simulink model "SimulinkAnalysisofCheetahTail"  (R2022a)
settings: Solver=ode4  StartTime=0.0  StopTime=1.5  FixedStep=0.001  RelTol=1e-3
undefined symbols (not defined in the file): B_cg_H, B_con_H, B_con_L, bar_len, cd_table, Cf, cl_table, g, gear_ratio, int_point_bar, int_point_tail, ITail, M_add, M_cg_H, M_cg_L, M_cg_W, Mb, Mm, Mt, psi3, rho, T_cg_H, T_fur_gap, T_length, T_width_major, T_width_minor, th2_initial, torque_constant, uncertainty_Forces, uncertainty_Position, Vf, windspeed
(part 16 of 21)

== matlab function SimulinkAnalysisofCheetahTail/Model/Forces/NonConstraintForceMatrix_tail_5 ==
  data: B_con_H parameter; B_con_L parameter; Cd input; Cl input; M_cg_H parameter; M_cg_L parameter; M_cg_W parameter; T_fur_gap parameter; T_length parameter; T_width_major parameter; T_width_minor parameter; area_tail_5_drag input; bar_len parameter; int_point_tail input; psi3 parameter; rho parameter; windspeed parameter; q input; dq input; ddq input; Q_tail_5 output
function Q_tail_5 = NonConstraintForceMatrix_tail_5(B_con_H,B_con_L,Cd,Cl,M_cg_H,M_cg_L,M_cg_W,T_fur_gap,T_length,T_width_major,T_width_minor,area_tail_5_drag,bar_len,int_point_tail,psi3,rho,windspeed,q,dq,ddq)
%#codegen
[x,y,z,phi1,th1,psi1,phi2,th2] = deal(q(1),q(2),q(3),q(4),q(5),q(6),q(7),q(8));
[dx,dy,dz,dphi1,dth1,dpsi1,dphi2,dth2] = deal(dq(1),dq(2),dq(3),dq(4),dq(5),dq(6),dq(7),dq(8));
[ddx,ddy,ddz,ddphi1,ddth1,ddpsi1,ddphi2,ddth2] = deal(ddq(1),ddq(2),ddq(3),ddq(4),ddq(5),ddq(6),ddq(7),ddq(8));
%    This function was generated by the Symbolic Math Toolbox version 9.0.
%    17-Feb-2022 12:30:45

t2 = cos(phi1);
t3 = cos(phi2);
t4 = cos(psi1);
t5 = cos(psi3);
t6 = cos(th1);
t7 = cos(th2);
t8 = sin(phi1);
t9 = sin(phi2);
t10 = sin(psi1);
t11 = sin(psi3);
t12 = sin(th1);
t13 = sin(th2);
t14 = M_cg_L+x;
t15 = M_cg_W+y;
t16 = M_cg_H+z;
t19 = -int_point_tail;
t45 = T_length.*(9.0./1.0e+1);
t46 = bar_len.*(9.0./1.0e+1);
t47 = int_point_tail.*(9.0./1.0e+1);
t17 = B_con_L.*t6;
t18 = B_con_L.*t12;
t20 = t2.*t4;
t21 = t6.*t7;
t22 = t2.*t10;
t23 = t4.*t8;
t24 = t7.*t12;
t25 = t8.*t10;
t26 = t12.*t13;
t27 = B_con_H.*t2.*t6;
t29 = t6.*t14;
t30 = B_con_H.*t2.*t12;
t31 = B_con_H.*t6.*t8;
t34 = t12.*t14;
t38 = t6.*t9.*t13;
t40 = t6.*t10.*t13;
t42 = t8.*t9.*t12;
t48 = t2.*t3.*t6;
t49 = T_length+bar_len+t19;
t52 = t2.*t6.*t9;
t53 = t3.*t6.*t8;
t55 = t2.*t6.*t13;
t56 = t3.*t6.*t13;
t58 = t4.*t6.*t13;
t61 = t3.*t8.*t12;
t62 = t6.*t8.*t9;
t67 = t2.*t6.*t15;
t69 = t2.*t6.*t16;
t72 = t6.*t8.*t15;
t73 = t2.*t12.*t16;
t74 = t6.*t8.*t16;
t76 = t8.*t12.*t15;
t79 = -t47;
t105 = t5.*t6.*t8.*t13;
t111 = t6.*t8.*t11.*t13;
t28 = t4.*t17;
t32 = t4.*t18;
t33 = t10.*t17;
t35 = t10.*t18;
t36 = t2.*t26;
t37 = t3.*t26;
t39 = t9.*t24;
t41 = t10.*t24;
t43 = t12.*t25;
t44 = t9.*t26;
t50 = t2.*t21;
t51 = t4.*t21;
t54 = t12.*t20;
t57 = t3.*t24;
t59 = t4.*t24;
t60 = t10.*t21;
t63 = t12.*t22;
t64 = t12.*t23;
t65 = B_con_H.*t6.*t20;
t66 = t4.*t29;
t68 = B_con_H.*t6.*t22;
t70 = t4.*t34;
t71 = t10.*t29;
t75 = t10.*t34;
t77 = -t30;
t78 = -t31;
t81 = -t42;
t86 = t3.*t6.*t23;
t87 = t13.*t48;
t90 = t3.*t8.*t21;
t91 = t6.*t13.*t20;
t92 = t4.*t56;
t95 = t3.*t6.*t25;
t96 = t6.*t9.*t23;
t97 = t2.*t38;
t99 = t8.*t9.*t21;
t100 = t6.*t13.*t22;
t102 = t3.*t40;
t103 = t4.*t38;
t106 = t6.*t9.*t25;
t110 = t10.*t38;
t113 = -t58;
t116 = t6.*t16.*t20;
t117 = t6.*t15.*t23;
t118 = t6.*t16.*t22;
t119 = t6.*t15.*t25;
t120 = -t67;
t121 = -t72;
t122 = -t73;
t123 = -t74;
t124 = t3.*t20.*t21;
t125 = t3.*t21.*t22;
t126 = t9.*t20.*t21;
t127 = t9.*t21.*t22;
t133 = -t105;
t138 = t24+t55;
t226 = t45+t46+t79;
t80 = -t36;
t82 = -t43;
t83 = -t44;
t84 = t3.*t50;
t85 = t3.*t51;
t88 = t2.*t57;
t89 = t9.*t50;
t93 = t3.*t60;
t94 = t9.*t51;
t98 = t2.*t39;
t101 = t4.*t37;
t104 = t9.*t60;
t107 = -t50;
t108 = t10.*t37;
t109 = t4.*t44;
t112 = -t54;
t114 = -t60;
t115 = t10.*t44;
t129 = -t92;
t131 = -t99;
t136 = -t117;
t137 = -t119;
t139 = t22+t64;
t140 = t23+t63;
t141 = -t124;
t142 = -t125;
t149 = t5.*t138;
t153 = t11.*t138;
t157 = t52+t90;
t161 = t57+t87;
t162 = t59+t91;
t163 = t39+t97;
t164 = t41+t100;
t128 = -t84;
t130 = -t93;
t132 = -t104;
t134 = t4.*t83;
t135 = t10.*t83;
t143 = B_con_H.*t139;
t144 = B_con_H.*t140;
t145 = t21+t80;
t146 = t26+t107;
t147 = t20+t82;
t148 = t25+t112;
t150 = t3.*t139;
t151 = t3.*t140;
t152 = t7.*t140;
t154 = t9.*t139;
t155 = t9.*t140;
t156 = t13.*t140;
t165 = t15.*t139;
t166 = t15.*t140;
t167 = t16.*t139;
t168 = t16.*t140;
t174 = t5.*t13.*t139;
t176 = t11.*t13.*t139;
t184 = -t153;
t188 = t48+t131;
t189 = T_fur_gap.*t157;
t190 = T_fur_gap.*t161;
t191 = int_point_tail.*t157;
t192 = int_point_tail.*t161;
t199 = t5.*t162;
t200 = t11.*t162;
t201 = t5.*t163;
t202 = t5.*t164;
t203 = t11.*t163;
t204 = t11.*t164;
t228 = t38+t61+t98;
t231 = t56+t81+t88;
t232 = t53+t83+t89;
t266 = t96+t101+t141;
t268 = t106+t108+t142;
t295 = t157.*t226;
t296 = t161.*t226;
t158 = B_con_H.*t147;
t159 = B_con_H.*t148;
t160 = -t144;
t169 = t7.*t150;
t170 = t7.*t151;
t171 = t13.*t151;
t172 = t7.*t154;
t173 = t9.*t152;
t175 = t13.*t155;
t177 = t5.*t145;
t178 = t5.*t146;
t179 = t3.*t147;
t180 = t3.*t148;
t181 = t7.*t148;
t182 = t11.*t145;
t183 = t11.*t146;
t185 = t9.*t147;
t186 = t9.*t148;
t187 = t13.*t148;
t193 = t15.*t147;
t194 = t15.*t148;
t195 = -t166;
t196 = t16.*t147;
t197 = t16.*t148;
t198 = -t168;
t211 = t5.*t13.*t147;
t213 = t11.*t13.*t147;
t214 = -t176;
t220 = t5.*t188;
t221 = t11.*t188;
t222 = -t204;
t227 = t40+t152;
t229 = t114+t156;
t230 = t37+t62+t128;
t236 = t5.*t228;
t237 = t11.*t228;
t239 = T_fur_gap.*t231;
t240 = T_fur_gap.*t232;
t242 = int_point_tail.*t231;
t243 = int_point_tail.*t232;
t246 = -t5.*(t60-t156);
t249 = -t11.*(t60-t156);
t250 = t5.*t232;
t252 = t11.*t232;
t267 = t86+t126+t134;
t269 = t95+t127+t135;
t276 = T_fur_gap.*t266;
t277 = int_point_tail.*t266;
t278 = T_fur_gap.*t268;
t279 = int_point_tail.*t268;
t317 = t226.*t231;
t318 = t226.*t232;
t345 = t226.*t266;
t347 = t226.*t268;
t370 = t190+t192+t296;
t397 = t78+t120+t123+t189+t191+t295;
t205 = t7.*t179;
t206 = t7.*t180;
t207 = -t169;
t208 = t13.*t180;
t209 = t7.*t185;
t210 = t9.*t181;
t212 = t13.*t186;
t215 = -t177;
t216 = -t179;
t217 = -t183;
t218 = -t193;
t219 = -t194;
t225 = -t213;
t233 = t51+t187;
t234 = t5.*t227;
t235 = t11.*t227;
t238 = T_fur_gap.*t230;
t241 = int_point_tail.*t230;
t244 = t113+t181;
t251 = t12.*t230;
t254 = t130+t171;
t256 = t132+t175;
t257 = t2.*t6.*t230;
t258 = -t5.*(t58-t181);
t259 = t6.*t8.*t230;
t260 = -t11.*(t58-t181);
t262 = -T_fur_gap.*(t93-t171);
t264 = -int_point_tail.*(t93-t171);
t265 = t111+t220;
t270 = -t5.*(t104-t175);
t272 = -t11.*(t104-t175);
t274 = t5.*(t58-t181);
t280 = t133+t221;
t281 = t5.*t269;
t282 = t11.*t269;
t283 = t5.*t267;
t284 = t11.*t267;
t286 = t172+t180;
t288 = t178+t203;
t298 = -T_fur_gap.*(t169-t186);
t300 = -int_point_tail.*(t169-t186);
t302 = t149+t252;
t303 = t102+t170+t185;
t304 = t182+t236;
t308 = t184+t250;
t314 = t226.*t230;
t329 = -t12.*(t153-t250);
t335 = -t2.*t6.*(t153-t250);
t336 = -t6.*t8.*(t153-t250);
t342 = -t226.*(t93-t171);
t344 = t2.*t6.*(t153-t250);
t359 = -t226.*(t169-t186);
t395 = t240+t243+t318;
t396 = t230.*t370;
t401 = -t370.*(t153-t250);
t402 = t370.*(t153-t250);
t404 = -t230.*(t31+t67+t74-t189-t191-t295);
t412 = t17+t29+t76+t77+t122+t239+t242+t317;
t417 = (t153-t250).*(t31+t67+t74-t189-t191-t295);
t432 = t35+t68+t75+t118+t137+t278+t279+t347;
t433 = t32+t65+t70+t116+t136+t276+t277+t345;
t223 = -t205;
t224 = -t210;
t245 = t5.*t233;
t247 = t11.*t233;
t248 = -t234;
t253 = t85+t208;
t255 = t94+t212;
t273 = -t257;
t285 = t151+t209;
t287 = -t283;
t290 = t186+t207;
t292 = t5.*t286;
t294 = t11.*t286;
t301 = t201+t217;
t305 = T_fur_gap.*t303;
t306 = int_point_tail.*t303;
t307 = t129+t154+t206;
t310 = t215+t237;
t311 = t110+t173+t216;
t312 = t12.*t302;
t315 = t5.*t303.*windspeed;
t323 = t2.*t6.*t302;
t324 = t6.*t8.*t302;
t325 = t6.*t10.*t303;
t346 = t199+t284;
t348 = t202+t282;
t350 = t222+t281;
t352 = t140.*t303;
t353 = t235+t270;
t357 = t147.*t303;
t365 = t226.*t303;
t399 = t262+t264+t342;
t400 = t302.*t370;
t403 = t230.*t395;
t411 = t18+t27+t34+t69+t121+t238+t241+t314;
t413 = t302.*t395;
t414 = -t302.*(t31+t67+t74-t189-t191-t295);
t416 = -t395.*(t153-t250);
t418 = t395.*(t153-t250);
t424 = -t417;
t427 = -t303.*(T_fur_gap.*(t93-t171)+int_point_tail.*(t93-t171)+t226.*(t93-t171));
t431 = t303.*(T_fur_gap.*(t93-t171)+int_point_tail.*(t93-t171)+t226.*(t93-t171));
t439 = t230.*t412;
t452 = t302.*t412;
t453 = -t412.*(t153-t250);
t455 = t412.*(t153-t250);
t456 = t143+t167+t219+t298+t300+t359;
t462 = t303.*t432;
t261 = T_fur_gap.*t253;
t263 = int_point_tail.*t253;
t271 = t11.*t255;
t275 = t5.*t255;
t289 = t155+t223;
t291 = t5.*t285;
t293 = t11.*t285;
t309 = t103+t150+t224;
t313 = T_fur_gap.*t307;
t319 = int_point_tail.*t307;
t320 = T_fur_gap.*t311;
t322 = int_point_tail.*t311;
t327 = t5.*t311;
t330 = t11.*t311;
t332 = t11.*t307.*windspeed;
t333 = t19.*t307;
t334 = t4.*t6.*t307;
t337 = -t324;
t341 = t226.*t253;
t349 = t200+t287;
t351 = t174+t294;
t354 = t214+t292;
t356 = t139.*t307;
t360 = t248+t272;
t362 = t148.*t307;
t366 = t226.*t307;
t368 = t226.*t311;
t406 = -t403;
t422 = t157.*t411;
t423 = t161.*t411;
t428 = t231.*t411;
t429 = t232.*t411;
t434 = t5.*t230.*t411;
t435 = t11.*t230.*t411;
t441 = -t439;
t444 = t265.*t411;
t445 = -t411.*(t105-t221);
t447 = t288.*t411;
t448 = -t411.*(t183-t201);
t450 = t304.*t411;
t451 = -t411.*(t177-t237);
t454 = -t452;
t463 = t307.*t433;
t476 = t33+t71+t160+t198+t218+t305+t306+t365;
t481 = -t307.*(-t143-t167+t194+T_fur_gap.*(t169-t186)+int_point_tail.*(t169-t186)+t226.*(t169-t186));
t490 = t307.*(-t143-t167+t194+T_fur_gap.*(t169-t186)+int_point_tail.*(t169-t186)+t226.*(t169-t186));
t297 = T_fur_gap.*t289;
t299 = int_point_tail.*t289;
t316 = T_fur_gap.*t309;
t321 = int_point_tail.*t309;
t326 = t5.*t309;
t328 = t11.*t309;
t331 = -t313;
t338 = -t327;
t340 = -t332;
t343 = -t334;
t355 = t211+t293;
t358 = t226.*t289;
t361 = t225+t291;
t363 = t260+t275;
t364 = t271+t274;
t367 = t226.*t309;
t369 = -t366;
t372 = t246+t330;
t375 = t5.*windspeed.*(t330-t5.*(t60-t156));
t378 = t6.*t10.*(t330-t5.*(t60-t156));
t379 = -t5.*windspeed.*(t327+t11.*(t60-t156));
t384 = -t6.*t10.*(t327+t11.*(t60-t156));
t388 = t140.*(t330-t5.*(t60-t156));
t391 = t147.*(t330-t5.*(t60-t156));
t392 = -t140.*(t327+t11.*(t60-t156));
t394 = -t147.*(t327+t11.*(t60-t156));
t398 = t261+t263+t341;
t415 = t259+t356+t357;
t421 = t273+t352+t362;
t436 = -t428;
t437 = -t429;
t440 = -t435;
t443 = t320+t322+t368;
t446 = -t444;
t449 = -t447;
t459 = -(t330-t5.*(t60-t156)).*(T_fur_gap.*(t93-t171)+int_point_tail.*(t93-t171)+t226.*(t93-t171));
t461 = (t327+t11.*(t60-t156)).*(T_fur_gap.*(t93-t171)+int_point_tail.*(t93-t171)+t226.*(t93-t171));
t465 = -t463;
t492 = t432.*(t330-t5.*(t60-t156));
t496 = -t432.*(t327+t11.*(t60-t156));
t506 = -t476.*(t93-t171);
t507 = t476.*(t93-t171);
t508 = t268.*t476;
t510 = t289.*t476;
t518 = t5.*t303.*t476;
t519 = t11.*t303.*t476;
t520 = t311.*t476;
t522 = t348.*t476;
t524 = -t476.*(t204-t281);
t528 = t353.*t476;
t530 = -t476.*(t234+t11.*(t104-t175));
t532 = -t476.*(t213-t291);
t339 = -t328;
t371 = t247+t326;
t374 = t249+t338;
t385 = -t378;
t405 = t251+t325+t343;
t419 = ddy.*t415;
t420 = dy.*t415;
t425 = ddz.*t421;
t426 = dz.*t421;
t430 = t307.*t398;
t442 = t316+t321+t367;
t458 = t158+t195+t196+t297+t299+t358;
t464 = t303.*t443;
t478 = t28+t66+t159+t165+t197+t331+t333+t369;
t497 = -t492;
t500 = t443.*(t330-t5.*(t60-t156));
t502 = -t443.*(t327+t11.*(t60-t156));
t512 = -t510;
t521 = -t519;
t529 = t355.*t476;
t531 = -t528;
t373 = t245+t339;
t376 = t11.*t371.*windspeed;
t377 = t4.*t6.*t371;
t387 = t139.*t371;
t389 = t148.*t371;
t407 = ddx.*t405;
t408 = dx.*t405;
t438 = -t430;
t457 = t371.*t398;
t466 = t307.*t442;
t482 = t303.*t458;
t493 = t371.*t433;
t501 = t371.*t442;
t509 = t253.*t478;
t511 = t266.*t478;
t513 = -t371.*(-t143-t167+t194+T_fur_gap.*(t169-t186)+int_point_tail.*(t169-t186)+t226.*(t169-t186));
t515 = t458.*(t330-t5.*(t60-t156));
t516 = -t458.*(t327+t11.*(t60-t156));
t517 = -t478.*(t169-t186);
t523 = t309.*t478;
t525 = t5.*t307.*t478;
t526 = t11.*t307.*t478;
t533 = -t529;
t534 = t346.*t478;
t535 = t349.*t478;
t536 = t351.*t478;
t538 = -t478.*(t176-t292);
t539 = t478.*(t176-t292);
t540 = t363.*t478;
t541 = t364.*t478;
Q_tail_5 = ft_1({Cd,Cl,T_fur_gap,T_width_major,T_width_minor,area_tail_5_drag,ddphi1,ddphi2,ddth1,ddth2,ddx,ddy,ddz,dphi1,dphi2,dth1,dth2,dx,dy,dz,int_point_tail,rho,t10,t104,t105,t11,t12,t138,t139,t140,t143,t147,t148,t153,t156,t167,t169,t171,t175,t177,t186,t189,t191,t194,t2,t204,t213,t221,t226,t230,t232,t233,t234,t237,t250,t281,t291,t295,t302,t303,t307,t309,t31,t311,t312,t315,t323,t327,t329,t330,t332,t336,t337,t340,t344,t370,t371,t373,t375,t376,t377,t379,t384,t385,t387,t388,t389,t391,t392,t394,t395,t396,t398,t4,t400,t402,t403,t404,t406,t407,t408,t411,t412,t413,t414,t416,t417,t418,t419,t420,t422,t423,t424,t425,t426,t428,t429,t431,t432,t433,t434,t436,t437,t438,t439,t440,t441,t442,t443,t444,t445,t446,t447,t448,t449,t450,t451,t452,t453,t454,t455,t457,t458,t459,t461,t462,t463,t464,t465,t466,t476,t478,t481,t482,t49,t490,t492,t493,t496,t497,t5,t500,t501,t502,t507,t508,t509,t510,t511,t512,t513,t515,t516,t517,t518,t520,t521,t522,t523,t524,t525,t526,t529,t530,t531,t532,t533,t534,t535,t536,t538,t539,t540,t541,t6,t60,t67,t74,t8,t93,th2,windspeed});
end
function Q_tail_5 = ft_1(ct)
Cd = ct{1};
Cl = ct{2};
T_fur_gap = ct{3};
T_width_major = ct{4};
T_width_minor = ct{5};
area_tail_5_drag = ct{6};
ddphi1 = ct{7};
ddphi2 = ct{8};
ddth1 = ct{9};
ddth2 = ct{10};
ddx = ct{11};
ddy = ct{12};
ddz = ct{13};
dphi1 = ct{14};
dphi2 = ct{15};
dth1 = ct{16};
dth2 = ct{17};
dx = ct{18};
dy = ct{19};
dz = ct{20};
int_point_tail = ct{21};
rho = ct{22};
t10 = ct{23};
t104 = ct{24};
t105 = ct{25};
t11 = ct{26};
t12 = ct{27};
t138 = ct{28};
t139 = ct{29};
t140 = ct{30};
t143 = ct{31};
t147 = ct{32};
t148 = ct{33};
t153 = ct{34};
t156 = ct{35};
t167 = ct{36};
t169 = ct{37};
t171 = ct{38};
t175 = ct{39};
t177 = ct{40};
t186 = ct{41};
t189 = ct{42};
t191 = ct{43};
t194 = ct{44};
t2 = ct{45};
t204 = ct{46};
t213 = ct{47};
t221 = ct{48};
t226 = ct{49};
t230 = ct{50};
t232 = ct{51};
t233 = ct{52};
t234 = ct{53};
t237 = ct{54};
t250 = ct{55};
t281 = ct{56};
t291 = ct{57};
t295 = ct{58};
t302 = ct{59};
t303 = ct{60};
t307 = ct{61};
t309 = ct{62};
t31 = ct{63};
t311 = ct{64};
t312 = ct{65};
t315 = ct{66};
t323 = ct{67};
t327 = ct{68};
t329 = ct{69};
t330 = ct{70};
t332 = ct{71};
t336 = ct{72};
t337 = ct{73};
t340 = ct{74};
t344 = ct{75};
t370 = ct{76};
t371 = ct{77};
t373 = ct{78};
t375 = ct{79};
t376 = ct{80};
t377 = ct{81};
t379 = ct{82};
t384 = ct{83};
t385 = ct{84};
t387 = ct{85};
t388 = ct{86};
t389 = ct{87};
t391 = ct{88};
t392 = ct{89};
t394 = ct{90};
t395 = ct{91};
t396 = ct{92};
t398 = ct{93};
t4 = ct{94};
t400 = ct{95};
t402 = ct{96};
t403 = ct{97};
t404 = ct{98};
t406 = ct{99};
t407 = ct{100};
t408 = ct{101};
t411 = ct{102};
t412 = ct{103};
t413 = ct{104};
t414 = ct{105};
t416 = ct{106};
t417 = ct{107};
t418 = ct{108};
t419 = ct{109};
t420 = ct{110};
t422 = ct{111};
t423 = ct{112};
t424 = ct{113};
t425 = ct{114};
t426 = ct{115};
t428 = ct{116};
t429 = ct{117};
t431 = ct{118};
t432 = ct{119};
t433 = ct{120};
t434 = ct{121};
t436 = ct{122};
t437 = ct{123};
t438 = ct{124};
t439 = ct{125};
t440 = ct{126};
t441 = ct{127};
t442 = ct{128};
t443 = ct{129};
t444 = ct{130};
t445 = ct{131};
t446 = ct{132};
t447 = ct{133};
t448 = ct{134};
t449 = ct{135};
t450 = ct{136};
t451 = ct{137};
t452 = ct{138};
t453 = ct{139};
t454 = ct{140};
t455 = ct{141};
t457 = ct{142};
t458 = ct{143};
t459 = ct{144};
t461 = ct{145};
t462 = ct{146};
t463 = ct{147};
t464 = ct{148};
t465 = ct{149};
t466 = ct{150};
t476 = ct{151};
t478 = ct{152};
t481 = ct{153};
t482 = ct{154};
t49 = ct{155};
t490 = ct{156};
t492 = ct{157};
t493 = ct{158};
t496 = ct{159};
t497 = ct{160};
t5 = ct{161};
t500 = ct{162};
t501 = ct{163};
t502 = ct{164};
t507 = ct{165};
t508 = ct{166};
t509 = ct{167};
t510 = ct{168};
t511 = ct{169};
t512 = ct{170};
t513 = ct{171};
t515 = ct{172};
t516 = ct{173};
t517 = ct{174};
t518 = ct{175};
t520 = ct{176};
t521 = ct{177};
t522 = ct{178};
t523 = ct{179};
t524 = ct{180};
t525 = ct{181};
t526 = ct{182};
t529 = ct{183};
t530 = ct{184};
t531 = ct{185};
t532 = ct{186};
t533 = ct{187};
t534 = ct{188};
t535 = ct{189};
t536 = ct{190};
t538 = ct{191};
t539 = ct{192};
t540 = ct{193};
t541 = ct{194};
t6 = ct{195};
t60 = ct{196};
t67 = ct{197};
t74 = ct{198};
t8 = ct{199};
t93 = ct{200};
th2 = ct{201};
windspeed = ct{202};
t380 = t11.*t373.*windspeed;
t381 = -t376;
t382 = t4.*t6.*t373;
t383 = -t377;
t390 = t139.*t373;
t393 = t148.*t373;
t409 = -t407;
t410 = -t408;
t460 = t373.*t398;
t467 = -t466;
t472 = -ddx.*(t377+t12.*(t153-t250)+t6.*t10.*(t327+t11.*(t60-t156)));
t473 = -dx.*(t377+t12.*(t153-t250)+t6.*t10.*(t327+t11.*(t60-t156)));
t474 = ddx.*(t377+t12.*(t153-t250)+t6.*t10.*(t327+t11.*(t60-t156)));
t475 = dx.*(t377+t12.*(t153-t250)+t6.*t10.*(t327+t11.*(t60-t156)));
t479 = t336+t387+t394;
t485 = -ddy.*(-t387+t147.*(t327+t11.*(t60-t156))+t6.*t8.*(t153-t250));
t487 = -dy.*(-t387+t147.*(t327+t11.*(t60-t156))+t6.*t8.*(t153-t250));
t489 = t344+t389+t392;
t491 = -t482;
t498 = t373.*t433;
t499 = -t493;
t503 = t373.*t442;
t504 = -t501;
t514 = -t373.*(-t143-t167+t194+T_fur_gap.*(t169-t186)+int_point_tail.*(t169-t186)+t226.*(t169-t186));
t527 = -t525;
t537 = -t535;
t542 = -t541;
t543 = t396+t423+t431+t438+t507+t509;
t548 = t436+t441+t462+t465+t508+t511;
t549 = -ddth1.*(t428+t439-t462+t463-t508-t511);
t550 = -dth1.*(t428+t439-t462+t463-t508-t511);
t552 = t402+t448+t457+t461+t531+t540;
t554 = -ddphi2.*(t403+t429-t464+t466-t520-t523);
t555 = -dphi2.*(t403+t429-t464+t466-t520-t523);
t561 = -ddphi1.*(-t422+t481+t482+t510+t230.*(t31+t67+t74-t189-t191-t295)+t478.*(t169-t186));
t562 = -dphi1.*(-t422+t481+t482+t510+t230.*(t31+t67+t74-t189-t191-t295)+t478.*(t169-t186));
t563 = ddphi1.*(-t422+t481+t482+t510+t230.*(t31+t67+t74-t189-t191-t295)+t478.*(t169-t186));
t564 = dphi1.*(-t422+t481+t482+t510+t230.*(t31+t67+t74-t189-t191-t295)+t478.*(t169-t186));
t569 = -ddphi2.*(t416-t434+t501-t518+t525+t443.*(t327+t11.*(t60-t156)));
t570 = -dphi2.*(t416-t434+t501-t518+t525+t443.*(t327+t11.*(t60-t156)));
t577 = -ddth1.*(-t450+t453+t493+t535+t432.*(t327+t11.*(t60-t156))+t476.*(t204-t281));
t578 = -dth1.*(-t450+t453+t493+t535+t432.*(t327+t11.*(t60-t156))+t476.*(t204-t281));
t580 = -ddphi1.*(-t515+t529-t536+t302.*(t31+t67+t74-t189-t191-t295)+t411.*(t105-t221)+t373.*(-t143-t167+t194+T_fur_gap.*(t169-t186)+int_point_tail.*(t169-t186)+t226.*(t169-t186)));
t581 = -dphi1.*(-t515+t529-t536+t302.*(t31+t67+t74-t189-t191-t295)+t411.*(t105-t221)+t373.*(-t143-t167+t194+T_fur_gap.*(t169-t186)+int_point_tail.*(t169-t186)+t226.*(t169-t186)));
t582 = t424+t446+t513+t516+t532+t539;
t583 = -ddphi1.*(t417+t444+t538+t458.*(t327+t11.*(t60-t156))+t476.*(t213-t291)+t371.*(-t143-t167+t194+T_fur_gap.*(t169-t186)+int_point_tail.*(t169-t186)+t226.*(t169-t186)));
t584 = -dphi1.*(t417+t444+t538+t458.*(t327+t11.*(t60-t156))+t476.*(t213-t291)+t371.*(-t143-t167+t194+T_fur_gap.*(t169-t186)+int_point_tail.*(t169-t186)+t226.*(t169-t186)));
t386 = -t380;
t468 = t312+t382+t385;
t471 = t329+t383+t384;
t477 = t323+t388+t393;
t480 = t337+t390+t391;
t494 = ddz.*t489;
t495 = dz.*t489;
t505 = -t503;
t544 = ddth2.*t543;
t545 = dth2.*t543;
t551 = t406+t437+t464+t467+t520+t523;
t553 = t400+t449+t459+t460+t530+t542;
t556 = ddth2.*t552;
t557 = -ddth2.*(-t400+t447-t460+t541+t476.*(t234+t11.*(t104-t175))+(t330-t5.*(t60-t156)).*(T_fur_gap.*(t93-t171)+int_point_tail.*(t93-t171)+t226.*(t93-t171)));
t558 = dth2.*t552;
t559 = -dth2.*(-t400+t447-t460+t541+t476.*(t234+t11.*(t104-t175))+(t330-t5.*(t60-t156)).*(T_fur_gap.*(t93-t171)+int_point_tail.*(t93-t171)+t226.*(t93-t171)));
t560 = t404+t422+t490+t491+t512+t517;
t568 = t418+t434+t502+t504+t518+t527;
t571 = t451+t454+t497+t498+t522+t534;
t572 = -ddth1.*(t452+t492-t498-t522-t534+t411.*(t177-t237));
t573 = -dth1.*(t452+t492-t498-t522-t534+t411.*(t177-t237));
t574 = ddth1.*(t452+t492-t498-t522-t534+t411.*(t177-t237));
t575 = dth1.*(t452+t492-t498-t522-t534+t411.*(t177-t237));
t576 = t450+t455+t496+t499+t524+t537;
t579 = t414+t445+t514+t515+t533+t536;
t469 = ddx.*t468;
t470 = dx.*t468;
t483 = ddz.*t477;
t484 = dz.*t477;
t486 = ddy.*t480;
t488 = dy.*t480;
t546 = -t544;
t547 = -t545;
t565 = t413+t440+t500+t505+t521+t526;
t594 = t474+t485+t494+t556+t569+t577+t583;
t600 = t379+t381+t475+t487+t495+t558+t570+t578+t584;
t602 = -1.0./(t376+t473-t495-t558+dy.*(-t387+t147.*(t327+t11.*(t60-t156))+t6.*t8.*(t153-t250))+dphi2.*(t416-t434+t501-t518+t525+t443.*(t327+t11.*(t60-t156)))+dphi1.*(t417+t444+t538+t458.*(t327+t11.*(t60-t156))+t476.*(t213-t291)+t371.*(-t143-t167+t194+T_fur_gap.*(t169-t186)+int_point_tail.*(t169-t186)+t226.*(t169-t186)))+dth1.*(-t450+t453+t493+t535+t432.*(t327+t11.*(t60-t156))+t476.*(t204-t281))+t5.*windspeed.*(t327+t11.*(t60-t156)));
et1 = 1.0./(t376+t473-t495-t558+dy.*(-t387+t147.*(t327+t11.*(t60-t156))+t6.*t8.*(t153-t250))+dphi2.*(t416-t434+t501-t518+t525+t443.*(t327+t11.*(t60-t156)))+dphi1.*(t417+t444+t538+t458.*(t327+t11.*(t60-t156))+t476.*(t213-t291)+t371.*(-t143-t167+t194+T_fur_gap.*(t169-t186)+int_point_tail.*(t169-t186)+t226.*(t169-t186)))+dth1.*(-t450+t453+t493+t535+t432.*(t327+t11.*(t60-t156))+t476.*(t204-t281))+t5.*windspeed.*(t327+t11.*(t60-t156)));
et2 = -t315+t332+t408-t420-t426+t545+t562+dphi2.*(t403+t429-t464+t466-t520-t523)+dth1.*(t428+t439-t462+t463-t508-t511);
t604 = et1.*et2;
t566 = ddphi2.*t565;
t567 = dphi2.*t565;
t585 = t409+t419+t425+t546+t549+t554+t563;
t588 = t315+t340+t410+t420+t426+t547+t550+t555+t564;
t595 = abs(t594);
t601 = abs(t600);
t605 = atan(t604);
t586 = abs(t585);
t589 = abs(t588);
t591 = t469+t483+t486+t557+t566+t574+t580;
t596 = t595.^2;
t597 = t375+t386+t470+t484+t488+t559+t567+t575+t581;
t603 = t601.^2;
t606 = -t605;
t587 = t586.^2;
t590 = t589.^2;
t592 = abs(t591);
t598 = abs(t597);
t607 = t606+th2;
t593 = t592.^2;
t599 = t598.^2;
t608 = cos(t607);
t609 = t587+t593+t596;
t612 = t590+t599+t603;
t610 = sqrt(t609);
t613 = sqrt(t612);
t615 = (Cd.*area_tail_5_drag.*rho.*t608.*t612)./2.0;
t611 = (T_width_major.*T_width_minor.*rho.*t49.*t610.*pi)./2.0e+1;
t614 = 1.0./t613;
t616 = Cl.*T_width_major.*T_width_minor.*rho.*t608.*t613.*pi.*(-t315+t332+t408-t420-t426+t545+t562+dphi2.*(t403+t429-t464+t466-t520-t523)+dth1.*(t428+t439-t462+t463-t508-t511)).*(-1.0./2.0);
t617 = Cl.*T_width_major.*T_width_minor.*rho.*t608.*t613.*pi.*(-t315+t332+t408-t420-t426+t545+t562+dphi2.*(t403+t429-t464+t466-t520-t523)+dth1.*(t428+t439-t462+t463-t508-t511)).*(-3.061616997868383e-17);
t618 = (Cl.*T_width_major.*T_width_minor.*rho.*t138.*t597.*t608.*t613.*pi)./2.0;
t619 = Cl.*T_width_major.*T_width_minor.*rho.*t608.*t613.*pi.*(t376+t473-t495-t558+dy.*(-t387+t147.*(t327+t11.*(t60-t156))+t6.*t8.*(t153-t250))+dphi2.*(t416-t434+t501-t518+t525+t443.*(t327+t11.*(t60-t156)))+dphi1.*(t417+t444+t538+t458.*(t327+t11.*(t60-t156))+t476.*(t213-t291)+t371.*(-t143-t167+t194+T_fur_gap.*(t169-t186)+int_point_tail.*(t169-t186)+t226.*(t169-t186)))+dth1.*(-t450+t453+t493+t535+t432.*(t327+t11.*(t60-t156))+t476.*(t204-t281))+t5.*windspeed.*(t327+t11.*(t60-t156))).*(-1.0./2.0);
t620 = (Cl.*T_width_major.*T_width_minor.*rho.*t233.*t597.*t608.*t613.*pi)./2.0;
t621 = Cl.*T_width_major.*T_width_minor.*rho.*t597.*t608.*t613.*pi.*(t60-t156).*(-1.0./2.0);
et3 = Cl.*T_width_major.*T_width_minor.*rho.*t608.*t613.*pi.*(t376+t473-t495-t558+dy.*(-t387+t147.*(t327+t11.*(t60-t156))+t6.*t8.*(t153-t250))+dphi2.*(t416-t434+t501-t518+t525+t443.*(t327+t11.*(t60-t156)))+dphi1.*(t417+t444+t538+t458.*(t327+t11.*(t60-t156))+t476.*(t213-t291)+t371.*(-t143-t167+t194+T_fur_gap.*(t169-t186)+int_point_tail.*(t169-t186)+t226.*(t169-t186)))+dth1.*(-t450+t453+t493+t535+t432.*(t327+t11.*(t60-t156))+t476.*(t204-t281))+t5.*windspeed.*(t327+t11.*(t60-t156)));
et4 = -3.061616997868383e-17;
t622 = et3.*et4;
et5 = Cl.*T_width_major.*T_width_minor.*rho.*t608.*t613.*pi.*(t376+t473-t495-t558+dy.*(-t387+t147.*(t327+t11.*(t60-t156))+t6.*t8.*(t153-t250))+dphi2.*(t416-t434+t501-t518+t525+t443.*(t327+t11.*(t60-t156)))+dphi1.*(t417+t444+t538+t458.*(t327+t11.*(t60-t156))+t476.*(t213-t291)+t371.*(-t143-t167+t194+T_fur_gap.*(t169-t186)+int_point_tail.*(t169-t186)+t226.*(t169-t186)))+dth1.*(-t450+t453+t493+t535+t432.*(t327+t11.*(t60-t156))+t476.*(t204-t281))+t5.*windspeed.*(t327+t11.*(t60-t156)));
et6 = 3.061616997868383e-17;
t623 = et5.*et6;
et7 = (Cl.*T_width_major.*T_width_minor.*rho.*t608.*t613.*pi.*(t376+t473-t495-t558+dy.*(-t387+t147.*(t327+t11.*(t60-t156))+t6.*t8.*(t153-t250))+dphi2.*(t416-t434+t501-t518+t525+t443.*(t327+t11.*(t60-t156)))+dphi1.*(t417+t444+t538+t458.*(t327+t11.*(t60-t156))+t476.*(t213-t291)+t371.*(-t143-t167+t194+T_fur_gap.*(t169-t186)+int_point_tail.*(t169-t186)+t226.*(t169-t186)))+dth1.*(-t450+t453+t493+t535+t432.*(t327+t11.*(t60-t156))+t476.*(t204-t281))+t5.*windspeed.*(t327+t11.*(t60-t156))))./2.0;
et8 = Cl.*T_width_major.*T_width_minor.*rho.*t608.*t613.*pi.*(-t315+t332+t408-t420-t426+t545+t562+dphi2.*(t403+t429-t464+t466-t520-t523)+dth1.*(t428+t439-t462+t463-t508-t511)).*3.061616997868383e-17;
t630 = -t230.*(et7+et8);
et9 = (Cl.*T_width_major.*T_width_minor.*rho.*t608.*t613.*pi.*(t376+t473-t495-t558+dy.*(-t387+t147.*(t327+t11.*(t60-t156))+t6.*t8.*(t153-t250))+dphi2.*(t416-t434+t501-t518+t525+t443.*(t327+t11.*(t60-t156)))+dphi1.*(t417+t444+t538+t458.*(t327+t11.*(t60-t156))+t476.*(t213-t291)+t371.*(-t143-t167+t194+T_fur_gap.*(t169-t186)+int_point_tail.*(t169-t186)+t226.*(t169-t186)))+dth1.*(-t450+t453+t493+t535+t432.*(t327+t11.*(t60-t156))+t476.*(t204-t281))+t5.*windspeed.*(t327+t11.*(t60-t156))))./2.0;
et10 = Cl.*T_width_major.*T_width_minor.*rho.*t608.*t613.*pi.*(-t315+t332+t408-t420-t426+t545+t562+dphi2.*(t403+t429-t464+t466-t520-t523)+dth1.*(t428+t439-t462+t463-t508-t511)).*3.061616997868383e-17;
t632 = t230.*(et9+et10);
et11 = (Cl.*T_width_major.*T_width_minor.*rho.*t608.*t613.*pi.*(t376+t473-t495-t558+dy.*(-t387+t147.*(t327+t11.*(t60-t156))+t6.*t8.*(t153-t250))+dphi2.*(t416-t434+t501-t518+t525+t443.*(t327+t11.*(t60-t156)))+dphi1.*(t417+t444+t538+t458.*(t327+t11.*(t60-t156))+t476.*(t213-t291)+t371.*(-t143-t167+t194+T_fur_gap.*(t169-t186)+int_point_tail.*(t169-t186)+t226.*(t169-t186)))+dth1.*(-t450+t453+t493+t535+t432.*(t327+t11.*(t60-t156))+t476.*(t204-t281))+t5.*windspeed.*(t327+t11.*(t60-t156))))./2.0;
et12 = Cl.*T_width_major.*T_width_minor.*rho.*t608.*t613.*pi.*(-t315+t332+t408-t420-t426+t545+t562+dphi2.*(t403+t429-t464+t466-t520-t523)+dth1.*(t428+t439-t462+t463-t508-t511)).*3.061616997868383e-17;
t633 = -t303.*(et11+et12);
et13 = (Cl.*T_width_major.*T_width_minor.*rho.*t608.*t613.*pi.*(t376+t473-t495-t558+dy.*(-t387+t147.*(t327+t11.*(t60-t156))+t6.*t8.*(t153-t250))+dphi2.*(t416-t434+t501-t518+t525+t443.*(t327+t11.*(t60-t156)))+dphi1.*(t417+t444+t538+t458.*(t327+t11.*(t60-t156))+t476.*(t213-t291)+t371.*(-t143-t167+t194+T_fur_gap.*(t169-t186)+int_point_tail.*(t169-t186)+t226.*(t169-t186)))+dth1.*(-t450+t453+t493+t535+t432.*(t327+t11.*(t60-t156))+t476.*(t204-t281))+t5.*windspeed.*(t327+t11.*(t60-t156))))./2.0;
et14 = Cl.*T_width_major.*T_width_minor.*rho.*t608.*t613.*pi.*(-t315+t332+t408-t420-t426+t545+t562+dphi2.*(t403+t429-t464+t466-t520-t523)+dth1.*(t428+t439-t462+t463-t508-t511)).*3.061616997868383e-17;
t634 = -t307.*(et13+et14);
t624 = t611+t615;
t628 = t617+t619;
t629 = t616+t623;
t625 = -t230.*t614.*t624.*(-t315+t332+t408-t420-t426+t545+t562+dphi2.*(t403+t429-t464+t466-t520-t523)+dth1.*(t428+t439-t462+t463-t508-t511));
t626 = -t303.*t614.*t624.*(-t315+t332+t408-t420-t426+t545+t562+dphi2.*(t403+t429-t464+t466-t520-t523)+dth1.*(t428+t439-t462+t463-t508-t511));
t627 = -t307.*t614.*t624.*(-t315+t332+t408-t420-t426+t545+t562+dphi2.*(t403+t429-t464+t466-t520-t523)+dth1.*(t428+t439-t462+t463-t508-t511));
t631 = t232.*t629;
t635 = t309.*t629;
t636 = t311.*t629;
t638 = t138.*t597.*t614.*t624;
t640 = t233.*t597.*t614.*t624;
t641 = -t597.*t614.*t624.*(t60-t156);
t642 = -t232.*t614.*t624.*(t376+t473-t495-t558+dy.*(-t387+t147.*(t327+t11.*(t60-t156))+t6.*t8.*(t153-t250))+dphi2.*(t416-t434+t501-t518+t525+t443.*(t327+t11.*(t60-t156)))+dphi1.*(t417+t444+t538+t458.*(t327+t11.*(t60-t156))+t476.*(t213-t291)+t371.*(-t143-t167+t194+T_fur_gap.*(t169-t186)+int_point_tail.*(t169-t186)+t226.*(t169-t186)))+dth1.*(-t450+t453+t493+t535+t432.*(t327+t11.*(t60-t156))+t476.*(t204-t281))+t5.*windspeed.*(t327+t11.*(t60-t156)));
t643 = -t309.*t614.*t624.*(t376+t473-t495-t558+dy.*(-t387+t147.*(t327+t11.*(t60-t156))+t6.*t8.*(t153-t250))+dphi2.*(t416-t434+t501-t518+t525+t443.*(t327+t11.*(t60-t156)))+dphi1.*(t417+t444+t538+t458.*(t327+t11.*(t60-t156))+t476.*(t213-t291)+t371.*(-t143-t167+t194+T_fur_gap.*(t169-t186)+int_point_tail.*(t169-t186)+t226.*(t169-t186)))+dth1.*(-t450+t453+t493+t535+t432.*(t327+t11.*(t60-t156))+t476.*(t204-t281))+t5.*windspeed.*(t327+t11.*(t60-t156)));
t644 = -t311.*t614.*t624.*(t376+t473-t495-t558+dy.*(-t387+t147.*(t327+t11.*(t60-t156))+t6.*t8.*(t153-t250))+dphi2.*(t416-t434+t501-t518+t525+t443.*(t327+t11.*(t60-t156)))+dphi1.*(t417+t444+t538+t458.*(t327+t11.*(t60-t156))+t476.*(t213-t291)+t371.*(-t143-t167+t194+T_fur_gap.*(t169-t186)+int_point_tail.*(t169-t186)+t226.*(t169-t186)))+dth1.*(-t450+t453+t493+t535+t432.*(t327+t11.*(t60-t156))+t476.*(t204-t281))+t5.*windspeed.*(t327+t11.*(t60-t156)));
t645 = t311.*t614.*t624.*(t376+t473-t495-t558+dy.*(-t387+t147.*(t327+t11.*(t60-t156))+t6.*t8.*(t153-t250))+dphi2.*(t416-t434+t501-t518+t525+t443.*(t327+t11.*(t60-t156)))+dphi1.*(t417+t444+t538+t458.*(t327+t11.*(t60-t156))+t476.*(t213-t291)+t371.*(-t143-t167+t194+T_fur_gap.*(t169-t186)+int_point_tail.*(t169-t186)+t226.*(t169-t186)))+dth1.*(-t450+t453+t493+t535+t432.*(t327+t11.*(t60-t156))+t476.*(t204-t281))+t5.*windspeed.*(t327+t11.*(t60-t156)));
t637 = -t635;
t639 = -t638;
t646 = t618+t631+t632;
t647 = t621+t633+t636;
t650 = t627+t640+t643;
t651 = t626+t641+t645;
t648 = t620+t634+t637;
t649 = t625+t639+t642;
et15 = t638+t232.*t614.*t624.*(t376+t473-t495-t558+dy.*(-t387+t147.*(t327+t11.*(t60-t156))+t6.*t8.*(t153-t250))+dphi2.*(t416-t434+t501-t518+t525+t443.*(t327+t11.*(t60-t156)))+dphi1.*(t417+t444+t538+t458.*(t327+t11.*(t60-t156))+t476.*(t213-t291)+t371.*(-t143-t167+t194+T_fur_gap.*(t169-t186)+int_point_tail.*(t169-t186)+t226.*(t169-t186)))+dth1.*(-t450+t453+t493+t535+t432.*(t327+t11.*(t60-t156))+t476.*(t204-t281))+t5.*windspeed.*(t327+t11.*(t60-t156)));
et16 = t230.*t614.*t624.*(-t315+t332+t408-t420-t426+t545+t562+dphi2.*(t403+t429-t464+t466-t520-t523)+dth1.*(t428+t439-t462+t463-t508-t511));
et17 = (Cl.*T_width_major.*T_width_minor.*rho.*t608.*t613.*pi.*(t376+t473-t495-t558+dy.*(-t387+t147.*(t327+t11.*(t60-t156))+t6.*t8.*(t153-t250))+dphi2.*(t416-t434+t501-t518+t525+t443.*(t327+t11.*(t60-t156)))+dphi1.*(t417+t444+t538+t458.*(t327+t11.*(t60-t156))+t476.*(t213-t291)+t371.*(-t143-t167+t194+T_fur_gap.*(t169-t186)+int_point_tail.*(t169-t186)+t226.*(t169-t186)))+dth1.*(-t450+t453+t493+t535+t432.*(t327+t11.*(t60-t156))+t476.*(t204-t281))+t5.*windspeed.*(t327+t11.*(t60-t156))))./2.0;
et18 = Cl.*T_width_major.*T_width_minor.*rho.*t608.*t613.*pi.*(-t315+t332+t408-t420-t426+t545+t562+dphi2.*(t403+t429-t464+t466-t520-t523)+dth1.*(t428+t439-t462+t463-t508-t511)).*3.061616997868383e-17;
et19 = (Cl.*T_width_major.*T_width_minor.*rho.*t608.*t613.*pi.*(t376+t473-t495-t558+dy.*(-t387+t147.*(t327+t11.*(t60-t156))+t6.*t8.*(t153-t250))+dphi2.*(t416-t434+t501-t518+t525+t443.*(t327+t11.*(t60-t156)))+dphi1.*(t417+t444+t538+t458.*(t327+t11.*(t60-t156))+t476.*(t213-t291)+t371.*(-t143-t167+t194+T_fur_gap.*(t169-t186)+int_point_tail.*(t169-t186)+t226.*(t169-t186)))+dth1.*(-t450+t453+t493+t535+t432.*(t327+t11.*(t60-t156))+t476.*(t204-t281))+t5.*windspeed.*(t327+t11.*(t60-t156))))./2.0;
et20 = Cl.*T_width_major.*T_width_minor.*rho.*t608.*t613.*pi.*(-t315+t332+t408-t420-t426+t545+t562+dphi2.*(t403+t429-t464+t466-t520-t523)+dth1.*(t428+t439-t462+t463-t508-t511)).*3.061616997868383e-17;
et21 = -t640+t309.*t614.*t624.*(t376+t473-t495-t558+dy.*(-t387+t147.*(t327+t11.*(t60-t156))+t6.*t8.*(t153-t250))+dphi2.*(t416-t434+t501-t518+t525+t443.*(t327+t11.*(t60-t156)))+dphi1.*(t417+t444+t538+t458.*(t327+t11.*(t60-t156))+t476.*(t213-t291)+t371.*(-t143-t167+t194+T_fur_gap.*(t169-t186)+int_point_tail.*(t169-t186)+t226.*(t169-t186)))+dth1.*(-t450+t453+t493+t535+t432.*(t327+t11.*(t60-t156))+t476.*(t204-t281))+t5.*windspeed.*(t327+t11.*(t60-t156)));
et22 = t307.*t614.*t624.*(-t315+t332+t408-t420-t426+t545+t562+dphi2.*(t403+t429-t464+t466-t520-t523)+dth1.*(t428+t439-t462+t463-t508-t511));
et23 = (Cl.*T_width_major.*T_width_minor.*rho.*t608.*t613.*pi.*(t376+t473-t495-t558+dy.*(-t387+t147.*(t327+t11.*(t60-t156))+t6.*t8.*(t153-t250))+dphi2.*(t416-t434+t501-t518+t525+t443.*(t327+t11.*(t60-t156)))+dphi1.*(t417+t444+t538+t458.*(t327+t11.*(t60-t156))+t476.*(t213-t291)+t371.*(-t143-t167+t194+T_fur_gap.*(t169-t186)+int_point_tail.*(t169-t186)+t226.*(t169-t186)))+dth1.*(-t450+t453+t493+t535+t432.*(t327+t11.*(t60-t156))+t476.*(t204-t281))+t5.*windspeed.*(t327+t11.*(t60-t156))))./2.0;
et24 = Cl.*T_width_major.*T_width_minor.*rho.*t608.*t613.*pi.*(-t315+t332+t408-t420-t426+t545+t562+dphi2.*(t403+t429-t464+t466-t520-t523)+dth1.*(t428+t439-t462+t463-t508-t511)).*3.061616997868383e-17;
et25 = -t640+t309.*t614.*t624.*(t376+t473-t495-t558+dy.*(-t387+t147.*(t327+t11.*(t60-t156))+t6.*t8.*(t153-t250))+dphi2.*(t416-t434+t501-t518+t525+t443.*(t327+t11.*(t60-t156)))+dphi1.*(t417+t444+t538+t458.*(t327+t11.*(t60-t156))+t476.*(t213-t291)+t371.*(-t143-t167+t194+T_fur_gap.*(t169-t186)+int_point_tail.*(t169-t186)+t226.*(t169-t186)))+dth1.*(-t450+t453+t493+t535+t432.*(t327+t11.*(t60-t156))+t476.*(t204-t281))+t5.*windspeed.*(t327+t11.*(t60-t156)));
et26 = t307.*t614.*t624.*(-t315+t332+t408-t420-t426+t545+t562+dphi2.*(t403+t429-t464+t466-t520-t523)+dth1.*(t428+t439-t462+t463-t508-t511));
et27 = (Cl.*T_width_major.*T_width_minor.*rho.*t608.*t613.*pi.*(t376+t473-t495-t558+dy.*(-t387+t147.*(t327+t11.*(t60-t156))+t6.*t8.*(t153-t250))+dphi2.*(t416-t434+t501-t518+t525+t443.*(t327+t11.*(t60-t156)))+dphi1.*(t417+t444+t538+t458.*(t327+t11.*(t60-t156))+t476.*(t213-t291)+t371.*(-t143-t167+t194+T_fur_gap.*(t169-t186)+int_point_tail.*(t169-t186)+t226.*(t169-t186)))+dth1.*(-t450+t453+t493+t535+t432.*(t327+t11.*(t60-t156))+t476.*(t204-t281))+t5.*windspeed.*(t327+t11.*(t60-t156))))./2.0;
et28 = Cl.*T_width_major.*T_width_minor.*rho.*t608.*t613.*pi.*(-t315+t332+t408-t420-t426+t545+t562+dphi2.*(t403+t429-t464+t466-t520-t523)+dth1.*(t428+t439-t462+t463-t508-t511)).*3.061616997868383e-17;
et29 = t638+t232.*t614.*t624.*(t376+t473-t495-t558+dy.*(-t387+t147.*(t327+t11.*(t60-t156))+t6.*t8.*(t153-t250))+dphi2.*(t416-t434+t501-t518+t525+t443.*(t327+t11.*(t60-t156)))+dphi1.*(t417+t444+t538+t458.*(t327+t11.*(t60-t156))+t476.*(t213-t291)+t371.*(-t143-t167+t194+T_fur_gap.*(t169-t186)+int_point_tail.*(t169-t186)+t226.*(t169-t186)))+dth1.*(-t450+t453+t493+t535+t432.*(t327+t11.*(t60-t156))+t476.*(t204-t281))+t5.*windspeed.*(t327+t11.*(t60-t156)));
et30 = t230.*t614.*t624.*(-t315+t332+t408-t420-t426+t545+t562+dphi2.*(t403+t429-t464+t466-t520-t523)+dth1.*(t428+t439-t462+t463-t508-t511));
et31 = (Cl.*T_width_major.*T_width_minor.*rho.*t608.*t613.*pi.*(t376+t473-t495-t558+dy.*(-t387+t147.*(t327+t11.*(t60-t156))+t6.*t8.*(t153-t250))+dphi2.*(t416-t434+t501-t518+t525+t443.*(t327+t11.*(t60-t156)))+dphi1.*(t417+t444+t538+t458.*(t327+t11.*(t60-t156))+t476.*(t213-t291)+t371.*(-t143-t167+t194+T_fur_gap.*(t169-t186)+int_point_tail.*(t169-t186)+t226.*(t169-t186)))+dth1.*(-t450+t453+t493+t535+t432.*(t327+t11.*(t60-t156))+t476.*(t204-t281))+t5.*windspeed.*(t327+t11.*(t60-t156))))./2.0;
et32 = Cl.*T_width_major.*T_width_minor.*rho.*t608.*t613.*pi.*(-t315+t332+t408-t420-t426+t545+t562+dphi2.*(t403+t429-t464+t466-t520-t523)+dth1.*(t428+t439-t462+t463-t508-t511)).*3.061616997868383e-17;
et33 = -t640+t309.*t614.*t624.*(t376+t473-t495-t558+dy.*(-t387+t147.*(t327+t11.*(t60-t156))+t6.*t8.*(t153-t250))+dphi2.*(t416-t434+t501-t518+t525+t443.*(t327+t11.*(t60-t156)))+dphi1.*(t417+t444+t538+t458.*(t327+t11.*(t60-t156))+t476.*(t213-t291)+t371.*(-t143-t167+t194+T_fur_gap.*(t169-t186)+int_point_tail.*(t169-t186)+t226.*(t169-t186)))+dth1.*(-t450+t453+t493+t535+t432.*(t327+t11.*(t60-t156))+t476.*(t204-t281))+t5.*windspeed.*(t327+t11.*(t60-t156)));
et34 = t307.*t614.*t624.*(-t315+t332+t408-t420-t426+t545+t562+dphi2.*(t403+t429-t464+t466-t520-t523)+dth1.*(t428+t439-t462+t463-t508-t511));
et35 = (Cl.*T_width_major.*T_width_minor.*rho.*t608.*t613.*pi.*(t376+t473-t495-t558+dy.*(-t387+t147.*(t327+t11.*(t60-t156))+t6.*t8.*(t153-t250))+dphi2.*(t416-t434+t501-t518+t525+t443.*(t327+t11.*(t60-t156)))+dphi1.*(t417+t444+t538+t458.*(t327+t11.*(t60-t156))+t476.*(t213-t291)+t371.*(-t143-t167+t194+T_fur_gap.*(t169-t186)+int_point_tail.*(t169-t186)+t226.*(t169-t186)))+dth1.*(-t450+t453+t493+t535+t432.*(t327+t11.*(t60-t156))+t476.*(t204-t281))+t5.*windspeed.*(t327+t11.*(t60-t156))))./2.0;
et36 = Cl.*T_width_major.*T_width_minor.*rho.*t608.*t613.*pi.*(-t315+t332+t408-t420-t426+t545+t562+dphi2.*(t403+t429-t464+t466-t520-t523)+dth1.*(t428+t439-t462+t463-t508-t511)).*3.061616997868383e-17;
et37 = t638+t232.*t614.*t624.*(t376+t473-t495-t558+dy.*(-t387+t147.*(t327+t11.*(t60-t156))+t6.*t8.*(t153-t250))+dphi2.*(t416-t434+t501-t518+t525+t443.*(t327+t11.*(t60-t156)))+dphi1.*(t417+t444+t538+t458.*(t327+t11.*(t60-t156))+t476.*(t213-t291)+t371.*(-t143-t167+t194+T_fur_gap.*(t169-t186)+int_point_tail.*(t169-t186)+t226.*(t169-t186)))+dth1.*(-t450+t453+t493+t535+t432.*(t327+t11.*(t60-t156))+t476.*(t204-t281))+t5.*windspeed.*(t327+t11.*(t60-t156)));
et38 = t230.*t614.*t624.*(-t315+t332+t408-t420-t426+t545+t562+dphi2.*(t403+t429-t464+t466-t520-t523)+dth1.*(t428+t439-t462+t463-t508-t511));
et39 = (Cl.*T_width_major.*T_width_minor.*rho.*t608.*t613.*pi.*(t376+t473-t495-t558+dy.*(-t387+t147.*(t327+t11.*(t60-t156))+t6.*t8.*(t153-t250))+dphi2.*(t416-t434+t501-t518+t525+t443.*(t327+t11.*(t60-t156)))+dphi1.*(t417+t444+t538+t458.*(t327+t11.*(t60-t156))+t476.*(t213-t291)+t371.*(-t143-t167+t194+T_fur_gap.*(t169-t186)+int_point_tail.*(t169-t186)+t226.*(t169-t186)))+dth1.*(-t450+t453+t493+t535+t432.*(t327+t11.*(t60-t156))+t476.*(t204-t281))+t5.*windspeed.*(t327+t11.*(t60-t156))))./2.0;
et40 = Cl.*T_width_major.*T_width_minor.*rho.*t608.*t613.*pi.*(-t315+t332+t408-t420-t426+t545+t562+dphi2.*(t403+t429-t464+t466-t520-t523)+dth1.*(t428+t439-t462+t463-t508-t511)).*3.061616997868383e-17;
et41 = (Cl.*T_width_major.*T_width_minor.*rho.*t608.*t613.*pi.*(t376+t473-t495-t558+dy.*(-t387+t147.*(t327+t11.*(t60-t156))+t6.*t8.*(t153-t250))+dphi2.*(t416-t434+t501-t518+t525+t443.*(t327+t11.*(t60-t156)))+dphi1.*(t417+t444+t538+t458.*(t327+t11.*(t60-t156))+t476.*(t213-t291)+t371.*(-t143-t167+t194+T_fur_gap.*(t169-t186)+int_point_tail.*(t169-t186)+t226.*(t169-t186)))+dth1.*(-t450+t453+t493+t535+t432.*(t327+t11.*(t60-t156))+t476.*(t204-t281))+t5.*windspeed.*(t327+t11.*(t60-t156))))./2.0;
et42 = Cl.*T_width_major.*T_width_minor.*rho.*t608.*t613.*pi.*(-t315+t332+t408-t420-t426+t545+t562+dphi2.*(t403+t429-t464+t466-t520-t523)+dth1.*(t428+t439-t462+t463-t508-t511)).*3.061616997868383e-17;
et43 = -t640+t309.*t614.*t624.*(t376+t473-t495-t558+dy.*(-t387+t147.*(t327+t11.*(t60-t156))+t6.*t8.*(t153-t250))+dphi2.*(t416-t434+t501-t518+t525+t443.*(t327+t11.*(t60-t156)))+dphi1.*(t417+t444+t538+t458.*(t327+t11.*(t60-t156))+t476.*(t213-t291)+t371.*(-t143-t167+t194+T_fur_gap.*(t169-t186)+int_point_tail.*(t169-t186)+t226.*(t169-t186)))+dth1.*(-t450+t453+t493+t535+t432.*(t327+t11.*(t60-t156))+t476.*(t204-t281))+t5.*windspeed.*(t327+t11.*(t60-t156)));
et44 = t307.*t614.*t624.*(-t315+t332+t408-t420-t426+t545+t562+dphi2.*(t403+t429-t464+t466-t520-t523)+dth1.*(t428+t439-t462+t463-t508-t511));
et45 = t638+t232.*t614.*t624.*(t376+t473-t495-t558+dy.*(-t387+t147.*(t327+t11.*(t60-t156))+t6.*t8.*(t153-t250))+dphi2.*(t416-t434+t501-t518+t525+t443.*(t327+t11.*(t60-t156)))+dphi1.*(t417+t444+t538+t458.*(t327+t11.*(t60-t156))+t476.*(t213-t291)+t371.*(-t143-t167+t194+T_fur_gap.*(t169-t186)+int_point_tail.*(t169-t186)+t226.*(t169-t186)))+dth1.*(-t450+t453+t493+t535+t432.*(t327+t11.*(t60-t156))+t476.*(t204-t281))+t5.*windspeed.*(t327+t11.*(t60-t156)));
et46 = t230.*t614.*t624.*(-t315+t332+t408-t420-t426+t545+t562+dphi2.*(t403+t429-t464+t466-t520-t523)+dth1.*(t428+t439-t462+t463-t508-t511));
et47 = t646.*(t31+t67+t74-t189-t191-t295)-(-t620+t635+t307.*(et39+et40)).*(-t143-t167+t194+T_fur_gap.*(t169-t186)+int_point_tail.*(t169-t186)+t226.*(t169-t186))-t458.*(t644+t303.*t614.*t624.*(-t315+t332+t408-t420-t426+t545+t562+dphi2.*(t403+t429-t464+t466-t520-t523)+dth1.*(t428+t439-t462+t463-t508-t511))+t597.*t614.*t624.*(t60-t156))+t458.*(-t636+t303.*(et41+et42)+(Cl.*T_width_major.*T_width_minor.*rho.*t597.*t608.*t613.*pi.*(t60-t156))./2.0);
et48 = (et43+et44).*(-t143-t167+t194+T_fur_gap.*(t169-t186)+int_point_tail.*(t169-t186)+t226.*(t169-t186))-(et45+et46).*(t31+t67+t74-t189-t191-t295);
et49 = t638+t232.*t614.*t624.*(t376+t473-t495-t558+dy.*(-t387+t147.*(t327+t11.*(t60-t156))+t6.*t8.*(t153-t250))+dphi2.*(t416-t434+t501-t518+t525+t443.*(t327+t11.*(t60-t156)))+dphi1.*(t417+t444+t538+t458.*(t327+t11.*(t60-t156))+t476.*(t213-t291)+t371.*(-t143-t167+t194+T_fur_gap.*(t169-t186)+int_point_tail.*(t169-t186)+t226.*(t169-t186)))+dth1.*(-t450+t453+t493+t535+t432.*(t327+t11.*(t60-t156))+t476.*(t204-t281))+t5.*windspeed.*(t327+t11.*(t60-t156)));
et50 = t230.*t614.*t624.*(-t315+t332+t408-t420-t426+t545+t562+dphi2.*(t403+t429-t464+t466-t520-t523)+dth1.*(t428+t439-t462+t463-t508-t511));
et51 = (Cl.*T_width_major.*T_width_minor.*rho.*t608.*t613.*pi.*(t376+t473-t495-t558+dy.*(-t387+t147.*(t327+t11.*(t60-t156))+t6.*t8.*(t153-t250))+dphi2.*(t416-t434+t501-t518+t525+t443.*(t327+t11.*(t60-t156)))+dphi1.*(t417+t444+t538+t458.*(t327+t11.*(t60-t156))+t476.*(t213-t291)+t371.*(-t143-t167+t194+T_fur_gap.*(t169-t186)+int_point_tail.*(t169-t186)+t226.*(t169-t186)))+dth1.*(-t450+t453+t493+t535+t432.*(t327+t11.*(t60-t156))+t476.*(t204-t281))+t5.*windspeed.*(t327+t11.*(t60-t156))))./2.0;
et52 = Cl.*T_width_major.*T_width_minor.*rho.*t608.*t613.*pi.*(-t315+t332+t408-t420-t426+t545+t562+dphi2.*(t403+t429-t464+t466-t520-t523)+dth1.*(t428+t439-t462+t463-t508-t511)).*3.061616997868383e-17;
et53 = -t640+t309.*t614.*t624.*(t376+t473-t495-t558+dy.*(-t387+t147.*(t327+t11.*(t60-t156))+t6.*t8.*(t153-t250))+dphi2.*(t416-t434+t501-t518+t525+t443.*(t327+t11.*(t60-t156)))+dphi1.*(t417+t444+t538+t458.*(t327+t11.*(t60-t156))+t476.*(t213-t291)+t371.*(-t143-t167+t194+T_fur_gap.*(t169-t186)+int_point_tail.*(t169-t186)+t226.*(t169-t186)))+dth1.*(-t450+t453+t493+t535+t432.*(t327+t11.*(t60-t156))+t476.*(t204-t281))+t5.*windspeed.*(t327+t11.*(t60-t156)));
et54 = t307.*t614.*t624.*(-t315+t332+t408-t420-t426+t545+t562+dphi2.*(t403+t429-t464+t466-t520-t523)+dth1.*(t428+t439-t462+t463-t508-t511));
et55 = (Cl.*T_width_major.*T_width_minor.*rho.*t608.*t613.*pi.*(t376+t473-t495-t558+dy.*(-t387+t147.*(t327+t11.*(t60-t156))+t6.*t8.*(t153-t250))+dphi2.*(t416-t434+t501-t518+t525+t443.*(t327+t11.*(t60-t156)))+dphi1.*(t417+t444+t538+t458.*(t327+t11.*(t60-t156))+t476.*(t213-t291)+t371.*(-t143-t167+t194+T_fur_gap.*(t169-t186)+int_point_tail.*(t169-t186)+t226.*(t169-t186)))+dth1.*(-t450+t453+t493+t535+t432.*(t327+t11.*(t60-t156))+t476.*(t204-t281))+t5.*windspeed.*(t327+t11.*(t60-t156))))./2.0;
et56 = Cl.*T_width_major.*T_width_minor.*rho.*t608.*t613.*pi.*(-t315+t332+t408-t420-t426+t545+t562+dphi2.*(t403+t429-t464+t466-t520-t523)+dth1.*(t428+t439-t462+t463-t508-t511)).*3.061616997868383e-17;
et57 = (Cl.*T_width_major.*T_width_minor.*rho.*t608.*t613.*pi.*(t376+t473-t495-t558+dy.*(-t387+t147.*(t327+t11.*(t60-t156))+t6.*t8.*(t153-t250))+dphi2.*(t416-t434+t501-t518+t525+t443.*(t327+t11.*(t60-t156)))+dphi1.*(t417+t444+t538+t458.*(t327+t11.*(t60-t156))+t476.*(t213-t291)+t371.*(-t143-t167+t194+T_fur_gap.*(t169-t186)+int_point_tail.*(t169-t186)+t226.*(t169-t186)))+dth1.*(-t450+t453+t493+t535+t432.*(t327+t11.*(t60-t156))+t476.*(t204-t281))+t5.*windspeed.*(t327+t11.*(t60-t156))))./2.0;
et58 = Cl.*T_width_major.*T_width_minor.*rho.*t608.*t613.*pi.*(-t315+t332+t408-t420-t426+t545+t562+dphi2.*(t403+t429-t464+t466-t520-t523)+dth1.*(t428+t439-t462+t463-t508-t511)).*3.061616997868383e-17;
et59 = -t640+t309.*t614.*t624.*(t376+t473-t495-t558+dy.*(-t387+t147.*(t327+t11.*(t60-t156))+t6.*t8.*(t153-t250))+dphi2.*(t416-t434+t501-t518+t525+t443.*(t327+t11.*(t60-t156)))+dphi1.*(t417+t444+t538+t458.*(t327+t11.*(t60-t156))+t476.*(t213-t291)+t371.*(-t143-t167+t194+T_fur_gap.*(t169-t186)+int_point_tail.*(t169-t186)+t226.*(t169-t186)))+dth1.*(-t450+t453+t493+t535+t432.*(t327+t11.*(t60-t156))+t476.*(t204-t281))+t5.*windspeed.*(t327+t11.*(t60-t156)));
et60 = t307.*t614.*t624.*(-t315+t332+t408-t420-t426+t545+t562+dphi2.*(t403+t429-t464+t466-t520-t523)+dth1.*(t428+t439-t462+t463-t508-t511));
et61 = (Cl.*T_width_major.*T_width_minor.*rho.*t608.*t613.*pi.*(t376+t473-t495-t558+dy.*(-t387+t147.*(t327+t11.*(t60-t156))+t6.*t8.*(t153-t250))+dphi2.*(t416-t434+t501-t518+t525+t443.*(t327+t11.*(t60-t156)))+dphi1.*(t417+t444+t538+t458.*(t327+t11.*(t60-t156))+t476.*(t213-t291)+t371.*(-t143-t167+t194+T_fur_gap.*(t169-t186)+int_point_tail.*(t169-t186)+t226.*(t169-t186)))+dth1.*(-t450+t453+t493+t535+t432.*(t327+t11.*(t60-t156))+t476.*(t204-t281))+t5.*windspeed.*(t327+t11.*(t60-t156))))./2.0;
et62 = Cl.*T_width_major.*T_width_minor.*rho.*t608.*t613.*pi.*(-t315+t332+t408-t420-t426+t545+t562+dphi2.*(t403+t429-t464+t466-t520-t523)+dth1.*(t428+t439-t462+t463-t508-t511)).*3.061616997868383e-17;
et63 = t638+t232.*t614.*t624.*(t376+t473-t495-t558+dy.*(-t387+t147.*(t327+t11.*(t60-t156))+t6.*t8.*(t153-t250))+dphi2.*(t416-t434+t501-t518+t525+t443.*(t327+t11.*(t60-t156)))+dphi1.*(t417+t444+t538+t458.*(t327+t11.*(t60-t156))+t476.*(t213-t291)+t371.*(-t143-t167+t194+T_fur_gap.*(t169-t186)+int_point_tail.*(t169-t186)+t226.*(t169-t186)))+dth1.*(-t450+t453+t493+t535+t432.*(t327+t11.*(t60-t156))+t476.*(t204-t281))+t5.*windspeed.*(t327+t11.*(t60-t156)));
et64 = t230.*t614.*t624.*(-t315+t332+t408-t420-t426+t545+t562+dphi2.*(t403+t429-t464+t466-t520-t523)+dth1.*(t428+t439-t462+t463-t508-t511));
et65 = (Cl.*T_width_major.*T_width_minor.*rho.*t608.*t613.*pi.*(t376+t473-t495-t558+dy.*(-t387+t147.*(t327+t11.*(t60-t156))+t6.*t8.*(t153-t250))+dphi2.*(t416-t434+t501-t518+t525+t443.*(t327+t11.*(t60-t156)))+dphi1.*(t417+t444+t538+t458.*(t327+t11.*(t60-t156))+t476.*(t213-t291)+t371.*(-t143-t167+t194+T_fur_gap.*(t169-t186)+int_point_tail.*(t169-t186)+t226.*(t169-t186)))+dth1.*(-t450+t453+t493+t535+t432.*(t327+t11.*(t60-t156))+t476.*(t204-t281))+t5.*windspeed.*(t327+t11.*(t60-t156))))./2.0;
et66 = Cl.*T_width_major.*T_width_minor.*rho.*t608.*t613.*pi.*(-t315+t332+t408-t420-t426+t545+t562+dphi2.*(t403+t429-t464+t466-t520-t523)+dth1.*(t428+t439-t462+t463-t508-t511)).*3.061616997868383e-17;
et67 = -t640+t309.*t614.*t624.*(t376+t473-t495-t558+dy.*(-t387+t147.*(t327+t11.*(t60-t156))+t6.*t8.*(t153-t250))+dphi2.*(t416-t434+t501-t518+t525+t443.*(t327+t11.*(t60-t156)))+dphi1.*(t417+t444+t538+t458.*(t327+t11.*(t60-t156))+t476.*(t213-t291)+t371.*(-t143-t167+t194+T_fur_gap.*(t169-t186)+int_point_tail.*(t169-t186)+t226.*(t169-t186)))+dth1.*(-t450+t453+t493+t535+t432.*(t327+t11.*(t60-t156))+t476.*(t204-t281))+t5.*windspeed.*(t327+t11.*(t60-t156)));
et68 = t307.*t614.*t624.*(-t315+t332+t408-t420-t426+t545+t562+dphi2.*(t403+t429-t464+t466-t520-t523)+dth1.*(t428+t439-t462+t463-t508-t511));
et69 = (Cl.*T_width_major.*T_width_minor.*rho.*t608.*t613.*pi.*(t376+t473-t495-t558+dy.*(-t387+t147.*(t327+t11.*(t60-t156))+t6.*t8.*(t153-t250))+dphi2.*(t416-t434+t501-t518+t525+t443.*(t327+t11.*(t60-t156)))+dphi1.*(t417+t444+t538+t458.*(t327+t11.*(t60-t156))+t476.*(t213-t291)+t371.*(-t143-t167+t194+T_fur_gap.*(t169-t186)+int_point_tail.*(t169-t186)+t226.*(t169-t186)))+dth1.*(-t450+t453+t493+t535+t432.*(t327+t11.*(t60-t156))+t476.*(t204-t281))+t5.*windspeed.*(t327+t11.*(t60-t156))))./2.0;
et70 = Cl.*T_width_major.*T_width_minor.*rho.*t608.*t613.*pi.*(-t315+t332+t408-t420-t426+t545+t562+dphi2.*(t403+t429-t464+t466-t520-t523)+dth1.*(t428+t439-t462+t463-t508-t511)).*3.061616997868383e-17;
et71 = t638+t232.*t614.*t624.*(t376+t473-t495-t558+dy.*(-t387+t147.*(t327+t11.*(t60-t156))+t6.*t8.*(t153-t250))+dphi2.*(t416-t434+t501-t518+t525+t443.*(t327+t11.*(t60-t156)))+dphi1.*(t417+t444+t538+t458.*(t327+t11.*(t60-t156))+t476.*(t213-t291)+t371.*(-t143-t167+t194+T_fur_gap.*(t169-t186)+int_point_tail.*(t169-t186)+t226.*(t169-t186)))+dth1.*(-t450+t453+t493+t535+t432.*(t327+t11.*(t60-t156))+t476.*(t204-t281))+t5.*windspeed.*(t327+t11.*(t60-t156)));
et72 = t230.*t614.*t624.*(-t315+t332+t408-t420-t426+t545+t562+dphi2.*(t403+t429-t464+t466-t520-t523)+dth1.*(t428+t439-t462+t463-t508-t511));
et73 = -t640+t309.*t614.*t624.*(t376+t473-t495-t558+dy.*(-t387+t147.*(t327+t11.*(t60-t156))+t6.*t8.*(t153-t250))+dphi2.*(t416-t434+t501-t518+t525+t443.*(t327+t11.*(t60-t156)))+dphi1.*(t417+t444+t538+t458.*(t327+t11.*(t60-t156))+t476.*(t213-t291)+t371.*(-t143-t167+t194+T_fur_gap.*(t169-t186)+int_point_tail.*(t169-t186)+t226.*(t169-t186)))+dth1.*(-t450+t453+t493+t535+t432.*(t327+t11.*(t60-t156))+t476.*(t204-t281))+t5.*windspeed.*(t327+t11.*(t60-t156)));
et74 = t307.*t614.*t624.*(-t315+t332+t408-t420-t426+t545+t562+dphi2.*(t403+t429-t464+t466-t520-t523)+dth1.*(t428+t439-t462+t463-t508-t511));
et75 = (Cl.*T_width_major.*T_width_minor.*rho.*t608.*t613.*pi.*(t376+t473-t495-t558+dy.*(-t387+t147.*(t327+t11.*(t60-t156))+t6.*t8.*(t153-t250))+dphi2.*(t416-t434+t501-t518+t525+t443.*(t327+t11.*(t60-t156)))+dphi1.*(t417+t444+t538+t458.*(t327+t11.*(t60-t156))+t476.*(t213-t291)+t371.*(-t143-t167+t194+T_fur_gap.*(t169-t186)+int_point_tail.*(t169-t186)+t226.*(t169-t186)))+dth1.*(-t450+t453+t493+t535+t432.*(t327+t11.*(t60-t156))+t476.*(t204-t281))+t5.*windspeed.*(t327+t11.*(t60-t156))))./2.0;
et76 = Cl.*T_width_major.*T_width_minor.*rho.*t608.*t613.*pi.*(-t315+t332+t408-t420-t426+t545+t562+dphi2.*(t403+t429-t464+t466-t520-t523)+dth1.*(t428+t439-t462+t463-t508-t511)).*3.061616997868383e-17;
et77 = (Cl.*T_width_major.*T_width_minor.*rho.*t608.*t613.*pi.*(t376+t473-t495-t558+dy.*(-t387+t147.*(t327+t11.*(t60-t156))+t6.*t8.*(t153-t250))+dphi2.*(t416-t434+t501-t518+t525+t443.*(t327+t11.*(t60-t156)))+dphi1.*(t417+t444+t538+t458.*(t327+t11.*(t60-t156))+t476.*(t213-t291)+t371.*(-t143-t167+t194+T_fur_gap.*(t169-t186)+int_point_tail.*(t169-t186)+t226.*(t169-t186)))+dth1.*(-t450+t453+t493+t535+t432.*(t327+t11.*(t60-t156))+t476.*(t204-t281))+t5.*windspeed.*(t327+t11.*(t60-t156))))./2.0;
et78 = Cl.*T_width_major.*T_width_minor.*rho.*t608.*t613.*pi.*(-t315+t332+t408-t420-t426+t545+t562+dphi2.*(t403+t429-t464+t466-t520-t523)+dth1.*(t428+t439-t462+t463-t508-t511)).*3.061616997868383e-17;
mt1 = [t12.*(et15+et16)-t12.*t646+t4.*t6.*(-t620+t635+t307.*(et17+et18))+t6.*t10.*(t644+t303.*t614.*t624.*(-t315+t332+t408-t420-t426+t545+t562+dphi2.*(t403+t429-t464+t466-t520-t523)+dth1.*(t428+t439-t462+t463-t508-t511))+t597.*t614.*t624.*(t60-t156))-t6.*t10.*(-t636+t303.*(et19+et20)+(Cl.*T_width_major.*T_width_minor.*rho.*t597.*t608.*t613.*pi.*(t60-t156))./2.0)-t4.*t6.*(et21+et22)];
mt2 = [-t147.*(t644+t303.*t614.*t624.*(-t315+t332+t408-t420-t426+t545+t562+dphi2.*(t403+t429-t464+t466-t520-t523)+dth1.*(t428+t439-t462+t463-t508-t511))+t597.*t614.*t624.*(t60-t156))+t147.*(-t636+t303.*(et23+et24)+(Cl.*T_width_major.*T_width_minor.*rho.*t597.*t608.*t613.*pi.*(t60-t156))./2.0)-t139.*(et25+et26)+t139.*(-t620+t635+t307.*(et27+et28))-t6.*t8.*(et29+et30)+t6.*t8.*t646];
mt3 = [-t140.*(t644+t303.*t614.*t624.*(-t315+t332+t408-t420-t426+t545+t562+dphi2.*(t403+t429-t464+t466-t520-t523)+dth1.*(t428+t439-t462+t463-t508-t511))+t597.*t614.*t624.*(t60-t156))+t140.*(-t636+t303.*(et31+et32)+(Cl.*T_width_major.*T_width_minor.*rho.*t597.*t608.*t613.*pi.*(t60-t156))./2.0)-t148.*(et33+et34)+t148.*(-t620+t635+t307.*(et35+et36))+t2.*t6.*(et37+et38)-t2.*t6.*t646;et47+et48];
mt4 = [t412.*(et49+et50)-t412.*t646-t432.*(t644+t303.*t614.*t624.*(-t315+t332+t408-t420-t426+t545+t562+dphi2.*(t403+t429-t464+t466-t520-t523)+dth1.*(t428+t439-t462+t463-t508-t511))+t597.*t614.*t624.*(t60-t156))+t432.*(-t636+t303.*(et51+et52)+(Cl.*T_width_major.*T_width_minor.*rho.*t597.*t608.*t613.*pi.*(t60-t156))./2.0)+t433.*(et53+et54)-t433.*(-t620+t635+t307.*(et55+et56))];
mt5 = [t478.*(t644+t303.*t614.*t624.*(-t315+t332+t408-t420-t426+t545+t562+dphi2.*(t403+t429-t464+t466-t520-t523)+dth1.*(t428+t439-t462+t463-t508-t511))+t597.*t614.*t624.*(t60-t156))-t478.*(-t636+t303.*(et57+et58)+(Cl.*T_width_major.*T_width_minor.*rho.*t597.*t608.*t613.*pi.*(t60-t156))./2.0)+t476.*(et59+et60)-t476.*(-t620+t635+t307.*(et61+et62))];
mt6 = [t395.*(et63+et64)-t395.*t646-t443.*(t644+t303.*t614.*t624.*(-t315+t332+t408-t420-t426+t545+t562+dphi2.*(t403+t429-t464+t466-t520-t523)+dth1.*(t428+t439-t462+t463-t508-t511))+t597.*t614.*t624.*(t60-t156))+t443.*(-t636+t303.*(et65+et66)+(Cl.*T_width_major.*T_width_minor.*rho.*t597.*t608.*t613.*pi.*(t60-t156))./2.0)+t442.*(et67+et68)-t442.*(-t620+t635+t307.*(et69+et70))];
mt7 = [t370.*(et71+et72)-t370.*t646-t398.*(et73+et74)+(t644+t303.*t614.*t624.*(-t315+t332+t408-t420-t426+t545+t562+dphi2.*(t403+t429-t464+t466-t520-t523)+dth1.*(t428+t439-t462+t463-t508-t511))+t597.*t614.*t624.*(t60-t156)).*(T_fur_gap.*(t93-t171)+int_point_tail.*(t93-t171)+t226.*(t93-t171))-(-t636+t303.*(et75+et76)+(Cl.*T_width_major.*T_width_minor.*rho.*t597.*t608.*t613.*pi.*(t60-t156))./2.0).*(T_fur_gap.*(t93-t171)+int_point_tail.*(t93-t171)+t226.*(t93-t171))+t398.*(-t620+t635+t307.*(et77+et78))];
Q_tail_5 = [mt1;mt2;mt3;mt4;mt5;mt6;mt7];
end
